simulink model "DPS368XTSA1"  (R2025a)
settings: Solver=VariableStepAuto  StartTime=0.0  StopTime=10.0  RelTol=1e-3
settings Model: Creator=slee7  LastModifiedBy=slee7

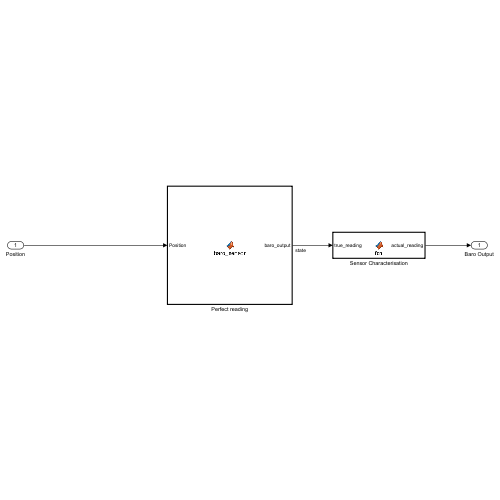
[thumbnail: Simulink's stored preview of the top-level diagram]
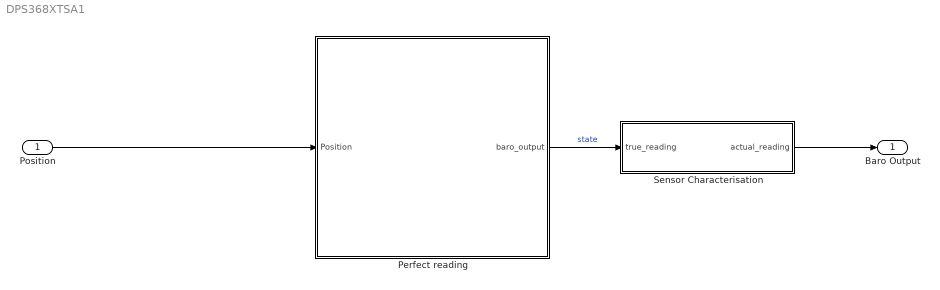
== system DPS368XTSA1 ==
  Position : Inport
  Perfect reading : MATLAB Function  TreatAsAtomicUnit=on
  Sensor Characterisation : MATLAB Function  TreatAsAtomicUnit=on
  Baro Output : Outport
  wires:
  Sensor Characterisation/1(actual_reading) -> Baro Output/1
  Position/1 -> Perfect reading/1(Position)
  Perfect reading/1(baro_output) -> Sensor Characterisation/1(true_reading)  "state"

== matlab function DPS368XTSA1/Sensor Characterisation ==
  data: true_reading input; actual_reading output
function actual_reading = fcn(true_reading)
    persistent b_previous

    dt = 0.0276; % Simulation Time Step for Standard 16x

    % Bias: Composite Bias = Const + Gauss-Markov Drift
    
        b_const = [-1.9576; -64.3354]; % Constant bias
    
        % Drift bias b_{k+1} &= e^{-\Delta t/ \tau} * b_k + \omega_k
        
        if isempty(b_previous)
            b_previous = [0; 0]; 
        end
    
        tau = [46.6667; 46.6601]; % time constant of drift
        q = [0.005501, 0.3838]; % variance on drift
    
        omega = sqrt(q) .* randn(2,1); % omega ~ N(0,q)
        
        phi = exp(-dt ./ tau);
        b_drift = phi .* b_previous + omega;

        b_previous = b_drift;
    
        composite_bias = b_const + b_drift; 

    % Noise: Gaussian (RMS resolution)  

        noise_std = [0.01; 0.35];      % [K_RMS; Pa_RMS]
    
        noise = noise_std .* randn(2,1); % noise ~ N(0,noise_variance)
    
    % Quantisation:

        quant_step = [0.01; 0.06]; % Quant Step: digital resolution
   

    % Reading Processing:

        actual_reading_continuous  = true_reading(:) + composite_bias + noise;

        actual_reading_quantised = quant_step * round(actual_reading_continuous/quant_step);

        actual_reading = actual_reading_quantised; 

end

% Currently Ignoring: 
% Scale_factor_error 
% Misalignment_error

== matlab function DPS368XTSA1/Perfect reading ==
  data: Position input; baro_output output
function baro_output = baro_sensor(Position)

% Constants
P_surface = 101325;        % Pa
T_surface = 288.15;        % K
M_0 = 28.9644;             % kg/kmol
R = 8.31446e3;             % N·m/(kmol·K)
g_0 = 9.80665;             % m/s^2
L = -0.0065;               % K/m
h_0 = 0;                   % m

% Height
h = Position(2);           % m

% Temperature model
Temperature = T_surface + (L * h-h_0);

% Barometric formula with lapse rate
exponent = (g_0 * M_0) / (R * L);
Pressure = P_surface * (T_surface / Temperature)^exponent;

baro_output = [Temperature, Pressure];
end
